simulink model "model_16_09_22"  (R2021a)
settings: Solver=FixedStepAuto  StartTime=0.0  StopTime=1370  FixedStep=0.01  RelTol=1e-3
values from neighbouring files (symbols this model uses):
  coord_0_ecef = [x_0_ecef, y_0_ecef, z_0_ecef]    [new_path_local_frame4_05_2022.m]
  dampPitchConst = 5    [Configuration_13_09_22FINESTRELLE.m]
  dampRollConst = 5    [Configuration_13_09_22FINESTRELLE.m]
  ECC = 0.0818191908426    [new_path_local_frame4_05_2022.m]
  FsGong = 8192    [matlabSounds.mat]
  FsHandel = 8192    [matlabSounds.mat]
  gainPitchTorque = -1000    [Configuration_13_09_22FINESTRELLE.m]
  gainRollTorque = -1000    [Configuration_13_09_22FINESTRELLE.m]
  indirect = 1    [Configuration_13_09_22FINESTRELLE.m]
  R_E = 6378137    [new_path_local_frame4_05_2022.m]
  RotationMatrix_NWU2ECEF = [-cos(lon0)*sin(lat0),  sin(lon0), cos(lon0)*cos(lat0) ... (first row only)    [new_path_local_frame4_05_2022.m]
  springPitchConst = 35    [Configuration_13_09_22FINESTRELLE.m]
  springRollConst = 35    [Configuration_13_09_22FINESTRELLE.m]
  timesPitch = 0.6    [Configuration_13_09_22FINESTRELLE.m]
  timesRoll = 0.6    [Configuration_13_09_22FINESTRELLE.m]
  yGong = [-0.00269844839217 -0.00449741398696 -0.00742073307848 -0.011018664268 -0.0128176298628 -0.0173150438498 -0.0222621992354 -0.0222621992354 -0.020013492242 -0.00921969867326 0.00449741398696 0.0101191814707 ... (42028 elements, 42028x1)]    [matlabSounds.mat]
  yHandel = [0 -0.00615680615681 -0.0750360750361 -0.0311688311688 0.00615680615681 0.0380952380952 0.0188552188552 -0.025012025012 -0.0311688311688 -0.0750360750361 -0.12582972583 -0.1443001443 ... (73113 elements, 73113x1)]    [matlabSounds.mat]
undefined symbols (not defined in the file or in its folder): DiscIntNeverNeededParam, f
libraries: cstblocks x7, simulink x6, instrumentlib x5
(part 1 of 2)
settings Model: SimulationMode=accelerator  Creator=vecluster  LastModifiedBy=LAR
settings SolverCC: AlgebraicLoopSolver=TrustRegion  MinimalZcImpactIntegration=on
settings DataIOCC: SaveFormat=StructureWithTime  SignalLoggingName=signals  ReturnWorkspaceOutputsName=ToWorkspace  LoggingToFile=on  LoggingFileName=logfile.mat
settings DebuggingCC: ArithmeticOperatorsInVariantConditions=warning
settings SFSimCC: CustomCodeUndefinedFunction=UseInterfaceOnly

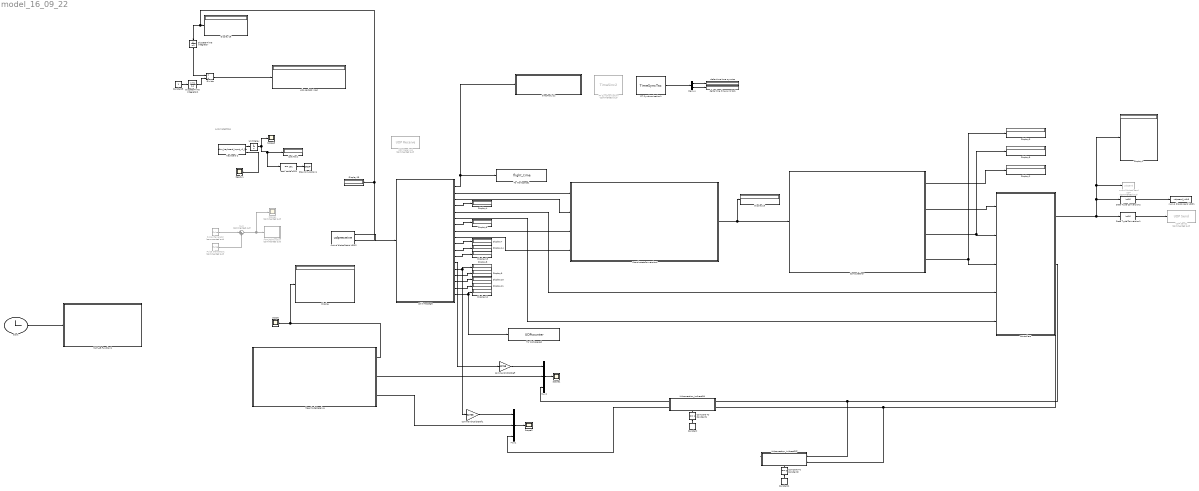
== system model_16_09_22 ==
  note: AutomatedStop
  Clock : Clock
  Compare To Constant1 : simulink/Logic and Bit Operations/Compare To Constant  relop===  const=1  OutDataTypeStr=boolean
  Compare To Constant2 : simulink/Logic and Bit Operations/Compare To Constant  relop===  const=0  OutDataTypeStr=boolean
  ComputeError : Subsystem
  Constant : Constant  Value=indirect  SampleTime=0.01
  Constant1 : Constant  Value=indirect  SampleTime=0.01
  Constant3 : Constant
  Controllers : Subsystem
  CoordinatesConversions : Subsystem
  Data Type Conversion1 : DataTypeConversion  OutDataTypeStr=int16
  Data Type Conversion2 : DataTypeConversion  OutDataTypeStr=int16
  Demux : Demux  Outputs=2
  Discrete-Time Integrator : DiscreteIntegrator  IntegratorMethod=Accumulation: Forward Euler  SampleTime=-1  ICPrevOutput=DiscIntNeverNeededParam  ICPrevScaledInput=DiscIntNeverNeededParam
  Discrete-Time Integrator1 : DiscreteIntegrator  InitialCondition=eps  SampleTime=-1  ICPrevOutput=DiscIntNeverNeededParam  ICPrevScaledInput=DiscIntNeverNeededParam
  Display{,1..16,23} (18 alike) : Display
  Divide : Product  Inputs=*/
  IHAcorrection_indirectON : Subsystem
  IHAcorrection_inidrectOFF : Subsystem
  Keyboard 2 : M-S-Function  FunctionName=sfun_keyboard_input_v1_2b  mask(Keyboard Input){}
      mask help: Keyboard Input
      mask Display: fprintf('Keyboard');
  Last Key1 : Display
  MATLAB Function : MATLAB Function  Commented=on  TreatAsAtomicUnit=on
  MATLAB Function1 : MATLAB Function  TreatAsAtomicUnit=on
  MagnitudeReceive : Subsystem
  Mux1 : Mux  Inputs=3
  Mux2 : Mux  Inputs=3
  Pulse Generator : DiscretePulseGenerator  Commented=on  PulseType=Time based  Period=1360  PulseWidth=0.01
  Pulse Generator1 : DiscretePulseGenerator  Commented=on  PulseType=Time based  Period=5  PulseWidth=0.1  PhaseDelay=1376
  RT Synchronization : S-Function  Commented=on  FunctionName=TimeSinc2  Parameters=st mf  SFunctionDeploymentMode=off  EnableBusSupport=off  mask(Pseudo-Real Time synchronization for Simulink Schemes){st=0.01, mf=200/140*200/255}
      mask prompts: st "Sample Time"; mf "Multiply factor"
      mask help:
      | This block synchronizes Simulink Simulation with RealTime.
      | The Real-Time versus Simulation-Time alignment is done every "Sample Time" seconds.
      | The Multiply Factor accelerates or slows real-Time: Multiply Factor=1 means real-time, Multiply Factor=2 means two times faster than real-time.
      | Use a Multiply Factor strictly > 0!!
      mask Display: disp(sprintf('RT Synchronization\n\nSample Time: %f\n Accelerator: %f',st,mf));
  RT Synchronization1 : S-Function  FunctionName=TimeSyncTsc  Parameters=st mf  SFunctionDeploymentMode=off  EnableBusSupport=off  mask(Pseudo-Real Time synchronization for Simulink Schemes){st=0.01, mf=1}
      mask prompts: st "Sample Time"; mf "Multiply factor"
      mask help:
      | This block synchronizes Simulink Simulation with RealTime.
      | The Real-Time versus Simulation-Time alignment is done every "Sample Time" seconds.
      | The Multiply Factor accelerates or slows real-Time: Multiply Factor=1 means real-time, Multiply Factor=2 means two times faster than real-time.
      | Use a Multiply Factor strictly > 0!!
      mask Display: disp(sprintf('RT Synchronization\n\nSample Time: %f\n Accelerator: %f',st,mf));
  Ready1 : Scope
  Scope{,1..3} (4 alike) : Scope
  Scope4 : Scope  Commented=on
  Stop Simulation1 : Stop
  Sum : Sum  Commented=on  Inputs=|++
  To Workspace1 : ToWorkspace  VariableName=flight_time  SaveFormat=Structure With Time  SampleTime=-1
  To Workspace2 : ToWorkspace  VariableName=UDPcounter  SaveFormat=Structure With Time  SampleTime=-1
  UDP Receive1 : instrumentlib/UDP Receive  Commented=on  Host=0.0.0.0  Port=1  LocalPort=6060  EnablePortSharing=on  GetLatestData=on  DataSize="[20   1]"  DataType=double  ASCIIFormatting=%f,  Terminator=LF  ByteOrder=LittleEndian  EnableBlockingMode=off  Timeout=100  SampleTime=0.01  LocalAddress=127.0.0.1
  UDP Send1 : instrumentlib/UDP Send  Commented=on  Host=192.168.51.103  Port=5347  LocalPort=-1  EnablePortSharing=on  ByteOrder=LittleEndian  OutputDatagramPacketSize=24  EnableBlockingMode=off  LocalAddress=0.0.0.0
  Unit Delay : UnitDelay  SampleTime=0.1  HasFrameUpgradeWarning=on
  ascii code of E1 : simulink/Logic and Bit Operations/Compare To Constant  relop===  const=101  OutDataTypeStr=boolean
  commandXstickDefl : Gain  Gain=32768
  commandXstickDefl1 : Gain  Gain=32768
  delta time time sync tsc : Display
  delta time time sync tsc1 : Display
  nuovo blocco send UDP : S-Function  Commented=on  FunctionName=udpsend  Parameters='127.0.0.1','192.168.51.103', 55555, 0.01  SFunctionDeploymentMode=off  EnableBusSupport=off
  nuovo blocco send UDP1 : S-Function  FunctionName=udpsend_int16  Parameters='127.0.0.1','192.168.51.103', 5347, 0.01  SFunctionDeploymentMode=off  EnableBusSupport=off
  nuovo blocco send UDP2 : S-Function  FunctionName=udpreceive  Parameters='127.0.0.1', 6060, 0.01, 20  SFunctionDeploymentMode=off  EnableBusSupport=off
  split message : MATLAB Function  TreatAsAtomicUnit=on
  timeAnalysis : Subsystem
  udp packets / sec : Display
  wires:
  Data Type Conversion1/1 -> UDP Send1/1  "StickCmd_INT16"
  CoordinatesConversions/1(plane_coord_nwu) -> Display23/1, ComputeError/1(plane_coord_nwu)  "plane_coord_nwu"
  split message/2(lat) -> CoordinatesConversions/1(lat)  "latRad"
  split message/3(lon) -> CoordinatesConversions/2(lon)  "lonRad"
  split message/8(coord_ecef_aerofly) -> CoordinatesConversions/3(aeroflyECEF)  "aeroflyECEF"
  split message/9(altitude) -> CoordinatesConversions/4(alt)  "altitude"
  ComputeError/2(intersection2path) -> Controllers/1(intesection2path)  "intesection2path"
  ComputeError/3(h) -> Display5/1, Controllers/2(h)  "h"
  ComputeError/4(s) -> Display3/1, Controllers/3(s)  "s"
  split message/5(roll) -> Controllers/4(rollAngle)  "roll"
  ComputeError/1(min_valid_index) -> Display2/1  "min_valid_index"
  Controllers/1(dataSend) -> Data Type Conversion2/1, nuovo blocco send UDP/1, Display1/1, Data Type Conversion1/1  "DataSend"
  split message/1(flight_time) -> timeAnalysis/1(flightTime), To Workspace1/1  "flightTime"
  split message/4(height) -> Display4/1  "height"
  split message/7(yaw) -> Display6/1  "yaw"
  split message/18(UDPcounter) -> Display12/1, To Workspace2/1  "UDPcounter"
  split message/14(aircraft_elevator) -> Display8/1, commandXstickDefl1/1  "elevator"
  split message/10(controls_roll_input) -> Display7/1  "control_roll_in"
  split message/11(controls_pitch_input) -> Display14/1  "control_pitch_in"
  split message/12(controls_yaw_input) -> Display13/1  "control_yaw_in"
  split message/6(pitch) -> Controllers/5(pitch)  "pitch"
  split message/15(aircraft_velocityX) -> Display9/1  "aircraftVelX"
  split message/16(aircraft_velocityY) -> Display10/1  "aircraftVelY"
  split message/17(aircraft_velocityZ) -> Display11/1  "aircraftVelZ"
  Mux2/1 -> Scope1/1
  commandXstickDefl/1 -> Mux2/1  "fromAileron2Command"
  Controllers/2(trimCorrectionRoll) -> IHAcorrection_inidrectOFF/1(trimCorrectionRoll), IHAcorrection_indirectON/1(trimCorrectionRoll)  "trimCorrectionsRoll"
  Controllers/3(trimCorrectionPitch) -> IHAcorrection_inidrectOFF/2(trimCorrectionPitch), IHAcorrection_indirectON/2(trimCorrectionPitch)  "trimCorrectionsPitch"
  IHAcorrection_indirectON/1(iha_correction_rollToSend) -> Mux2/3  "ihaCorrectionRollMagnitude"
  MagnitudeReceive/1(stickDeflectionVectorScaled) -> Display/1, Scope/1
  MagnitudeReceive/2(StickDeflRollReceived) -> Mux2/2  "StickDeflRollReceived"
  Constant/1 -> Compare To Constant1/1  "indirectON"
  Compare To Constant1/1 -> IHAcorrection_indirectON/Enable
  split message/13(aircraft_aileron) -> commandXstickDefl/1  "aileron"
  commandXstickDefl1/1 -> Mux1/1  "fromElevator2Command"
  MagnitudeReceive/3(StickDeflPitchReceived) -> Mux1/2  "StickDeflPitchReceived"
  IHAcorrection_indirectON/2(iha_correction_pitchToSend) -> Mux1/3  "ihaCorrectionPitchMagnitude"
  Mux1/1 -> Scope2/1
  Compare To Constant2/1 -> IHAcorrection_inidrectOFF/Enable
  Constant1/1 -> Compare To Constant2/1  "indirectOFF"
  IHAcorrection_inidrectOFF/1(iha_correction_rollToSend) -> ?
  Sum/1 -> MATLAB Function/1(start), Scope4/1  "audio"
  Pulse Generator1/1 -> Sum/2
  Pulse Generator/1 -> Sum/1
  ascii code of E1/1 -> Stop Simulation1/1
  Keyboard 2/2 -> Ready1/1
  Keyboard 2/1 -> Unit Delay/1
  RT Synchronization1/1 -> Demux/1  "TimeSyncTsc_output"
  Demux/1 -> delta time time sync tsc/1
  Unit Delay/1 -> ascii code of E1/1, Last Key1/1, Scope3/1
  nuovo blocco send UDP2/1 -> split message/1(u)  "UDPreceiveAerofly"
  nuovo blocco send UDP2/2 -> Discrete-Time Integrator/1, Display16/1, Display15/1  "UDPreceive1status"
  Discrete-Time Integrator/1 -> Divide/1
  Discrete-Time Integrator1/1 -> Divide/2
  Constant3/1 -> Discrete-Time Integrator1/1
  Divide/1 -> udp packets / sec/1  "packetsXsecondUDPreceive1"
  Demux/2 -> delta time time sync tsc1/1
  Data Type Conversion2/1 -> nuovo blocco send UDP1/1  "StickCmd_INT16"
  Clock/1 -> MATLAB Function1/1(start)  "simtime"

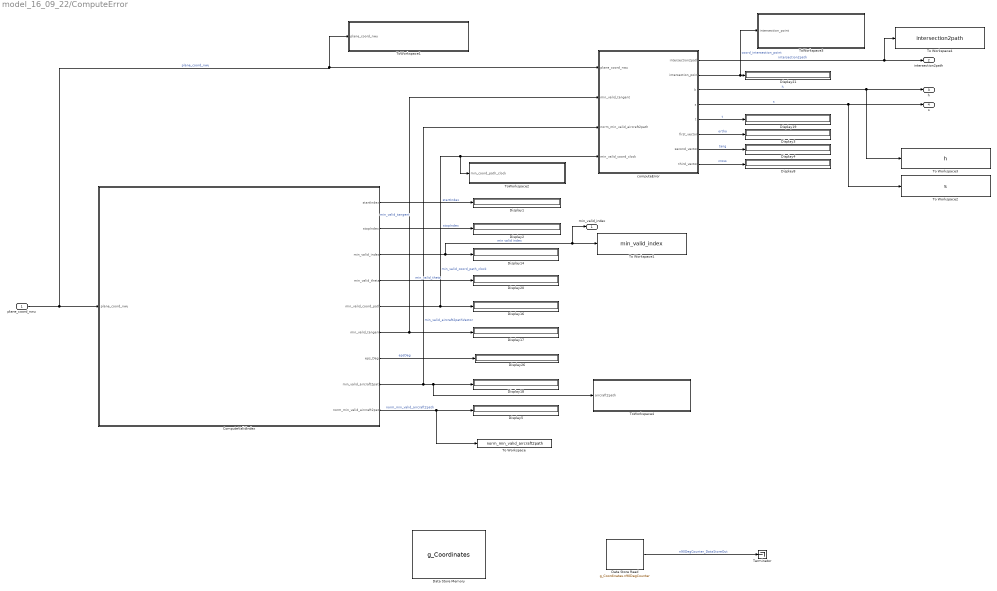
== system model_16_09_22/ComputeError ==
  plane_coord_nwu : Inport
  ComputeValidIndex : MATLAB Function  TreatAsAtomicUnit=on
  Data Store Memory : DataStoreMemory  DataStoreName=g_Coordinates  ReadBeforeWriteMsg=warning  WriteAfterWriteMsg=warning  WriteAfterReadMsg=warning  InitialValue=coord_clock_Struct  ShowAdditionalParam=off  OutDataTypeStr=Bus: ExperimentConfigAerofly
  Data Store Read : DataStoreRead  DataStoreName=g_Coordinates  DataStoreElements=g_Coordinates.n90DegCounter  IndexOptions=Index vector (dialog)  Indices=1  OutputSizes=1
  Display{1..5,8,14,16..21,26} (14 alike) : Display
  Terminator : Terminator
  To Workspace : ToWorkspace  VariableName=norm_min_valid_aircraft2path  SaveFormat=Structure With Time  SampleTime=-1
  To Workspace1 : ToWorkspace  VariableName=min_valid_index  SaveFormat=Structure With Time  SampleTime=-1
  To Workspace2 : ToWorkspace  VariableName=s  SaveFormat=Structure With Time  SampleTime=-1
  To Workspace3 : ToWorkspace  VariableName=h  SaveFormat=Structure With Time  SampleTime=-1
  To Workspace4 : ToWorkspace  VariableName=intersection2path  SaveFormat=Structure With Time  SampleTime=-1
  ToWorkspace1 : Subsystem
  ToWorkspace2 : Subsystem
  ToWorkspace3 : Subsystem
  ToWorkspace4 : Subsystem
  computeError : MATLAB Function  TreatAsAtomicUnit=on
  min_valid_index : Outport
  intersection2path : Outport  Port=2
  h : Outport  Port=3
  s : Outport  Port=4
  wires:
  computeError/1(intersection2path) -> To Workspace4/1, intersection2path/1  "intersection2path"
  ComputeValidIndex/7(eps_Deg) -> Display26/1  "epsDeg"
  computeError/6(first_vector) -> Display3/1  "ortho"
  ComputeValidIndex/4(min_valid_theta) -> Display20/1  "min_valid_theta"
  computeError/8(third_vector) -> Display8/1  "cross"
  computeError/7(second_vector) -> Display4/1  "tang"
  ComputeValidIndex/8(min_valid_aircraft2path) -> computeError/3(norm_min_valid_aircraft2path), ToWorkspace4/1(aircraft2path), Display18/1  "min_valid_aircraft2pathVector"
  ComputeValidIndex/6(min_valid_tangent) -> computeError/2(min_valid_tangent), Display17/1  "min_valid_tangent"
  computeError/5(t) -> Display19/1  "t"
  ComputeValidIndex/5(min_valid_coord_path) -> ToWorkspace2/1(min_coord_path_clock), computeError/4(min_valid_coord_clock), Display16/1  "min_valid_coord_path_clock"
  ComputeValidIndex/2(stopIndex) -> Display2/1  "stopIndex"
  computeError/2(intersection_point) -> ToWorkspace3/1(intersection_point), Display21/1  "coord_intersection_point"
  ComputeValidIndex/1(startIndex) -> Display1/1  "startIndex"
  ComputeValidIndex/3(min_valid_index) -> min_valid_index/1, To Workspace1/1, Display14/1  "min valid index"
  ComputeValidIndex/9(norm_min_valid_aircraft2path) -> Display5/1, To Workspace/1  "norm_min_valid_aircraft2path"
  Data Store Read/1 -> Terminator/1  "n90DegCounter_DataStoreOut"
  computeError/3(h) -> h/1, To Workspace3/1  "h"
  computeError/4(s) -> To Workspace2/1, s/1  "s"
  plane_coord_nwu/1 -> ComputeValidIndex/1(plane_coord_nwu), ToWorkspace1/1(plane_coord_nwu), computeError/1(plane_coord_nwu)  "plane_coord_nwu"

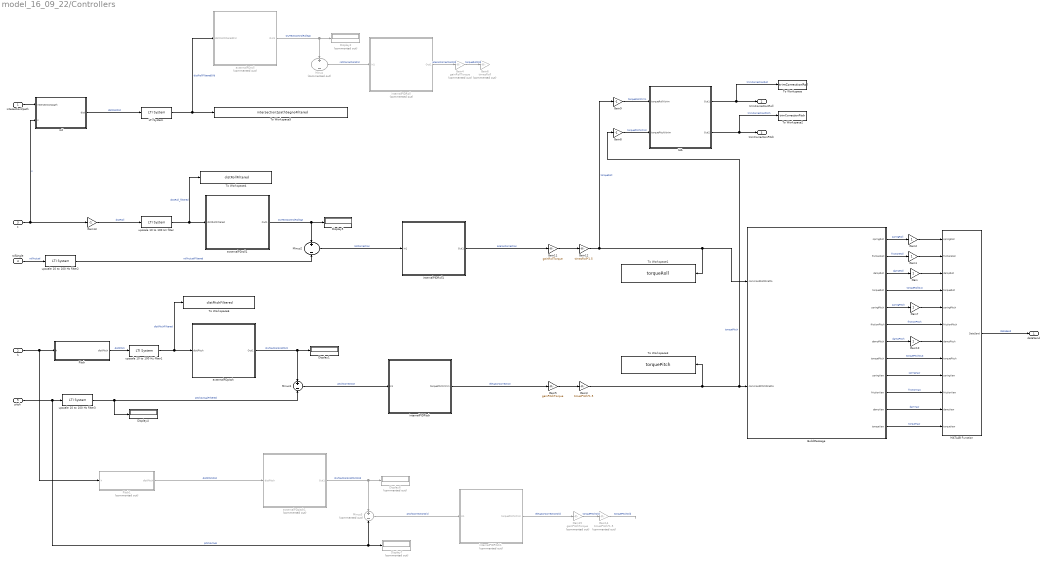
== system model_16_09_22/Controllers ==
  intesection2path : Inport
  h : Inport  Port=2
  s : Inport  Port=3
  rollAngle : Inport  Port=4
  pitch : Inport  Port=5
  BuildMessage : MATLAB Function  TreatAsAtomicUnit=on
  Display1 : Display
  Display2 : Display  Commented=on
  Display4 : Display
  Display5 : Display
  Display6 : Display  Commented=on
  Display7 : Display  Commented=on
  Gain{,1..2,7,10} (5 alike) : Gain
  Gain11 : Gain  Gain=gainRollTorque
  Gain12 : Gain  Gain=timesRoll*1.5
  Gain13 : Gain  Gain=-1
  Gain14 : Gain  Commented=on  Gain=timesPitch*1.5
  Gain15 : Gain  Commented=on  Gain=gainPitchTorque
  Gain3 : Gain  Gain=timesPitch*1.5
  Gain4 : Gain  Commented=on  Gain=gainRollTorque
  Gain5 : Gain  Gain=gainPitchTorque
  Gain6 : Gain  Commented=on  Gain=timesRoll
  Gain8 : Gain  Gain=-1
  Gain9 : Gain  Gain=-1
  IHA : Subsystem  TreatAsAtomicUnit=on
  LTI System : cstblocks/LTI System  sys=FILTER01  IC=[]
  MATLAB Function : MATLAB Function  TreatAsAtomicUnit=on
  Minus : Sum  Commented=on  Inputs=+-
  Minus1 : Sum  Inputs=+-
  Minus2 : Sum  Inputs=+-
  Minus3 : Sum  Commented=on  Inputs=+-
  Pitch : MATLAB Function  TreatAsAtomicUnit=on
  Pitch1 : MATLAB Function  Commented=on  TreatAsAtomicUnit=on
  To Workspace : ToWorkspace  VariableName=trimCorrectionRoll  SaveFormat=Structure With Time  SampleTime=-1
  To Workspace1 : ToWorkspace  VariableName=torqueRoll  SaveFormat=Structure With Time  SampleTime=-1
  To Workspace2 : ToWorkspace  VariableName=trimCorrectionPitch  SaveFormat=Structure With Time  SampleTime=-1
  To Workspace3 : ToWorkspace  VariableName=torquePitch  SaveFormat=Structure With Time  SampleTime=-1
  To Workspace4 : ToWorkspace  VariableName=distRollFiltered  SaveFormat=Structure With Time  SampleTime=-1
  To Workspace5 : ToWorkspace  VariableName=intersection2pathSegnoFiltered  SaveFormat=Structure With Time  SampleTime=-1
  To Workspace6 : ToWorkspace  VariableName=distPitchFiltered  SaveFormat=Structure With Time  SampleTime=-1
  externalPDpitch : Subsystem
  externalPDpitch1 : Subsystem  Commented=on
  externalPDroll : Subsystem  Commented=on
  externalPDroll1 : Subsystem
  internalPIDPitch : Subsystem
  internalPIDPitch1 : Subsystem  Commented=on
  internalPIDRoll : Subsystem  Commented=on
  internalPIDRoll1 : Subsystem
  roll : MATLAB Function  TreatAsAtomicUnit=on
  upscale 10 to 100 Hz filter{,1..3} (4 alike) : cstblocks/LTI System  sys=FILTER02  IC=[]
  dataSend : Outport
  trimCorrectionRoll : Outport  Port=2
  trimCorrectionPitch : Outport  Port=3
  wires:
  h/1 -> Pitch1/1(h), Pitch/1(h)
  s/1 -> Gain13/1, roll/2(s)  "s"
  Minus/1 -> internalPIDRoll/1(In1)  "rollCorrectionOld"
  Minus1/1 -> internalPIDPitch/1(In1)  "pitchCorrection"
  internalPIDPitch/1(torquePitchXtrim) -> Gain5/1  "elevatorCorrection"
  externalPDpitch/1(Out1) -> Display1/1, Minus1/1  "OUTextControlPitch"
  internalPIDRoll/1(Out1) -> Gain4/1  "aileronCorrectionOld"
  MATLAB Function/1(DataSend) -> dataSend/1  "DataSend"
  BuildMessage/3(dampRoll) -> Gain/1  "dampRoll"
  BuildMessage/4(torqueRoll) -> MATLAB Function/4(torqueRoll)  "torqueRollOut"
  BuildMessage/5(springPitch) -> Gain7/1  "springPitch"
  BuildMessage/6(frictionPitch) -> MATLAB Function/6(frictionPitch)  "frictionPitch"
  BuildMessage/7(dampPitch) -> Gain10/1  "dampPitch"
  BuildMessage/8(torquePitch) -> MATLAB Function/8(torquePitch)  "torquePitchOut"
  BuildMessage/9(springYaw) -> MATLAB Function/9(springYaw)  "springYaw"
  BuildMessage/10(frictionYaw) -> MATLAB Function/10(frictionYaw)  "frictionYaw"
  BuildMessage/11(dampYaw) -> MATLAB Function/11(dampYaw)  "damYaw"
  BuildMessage/12(torqueYaw) -> MATLAB Function/12(torqueYaw)  "torqueYaw"
  Pitch/1(distPitch) -> upscale 10 to 100 Hz filter1/1  "distPitch"
  externalPDroll/1(Out1) -> Minus/1, Display2/1  "OUTextControlRollSat"
  roll/1(dist) -> LTI System/1  "distRollOld"
  BuildMessage/2(frictionRoll) -> Gain1/1  "frictionRoll"
  BuildMessage/1(springRoll) -> Gain2/1  "springRoll"
  IHA/1(Out1) -> To Workspace/1, trimCorrectionRoll/1  "trimCorrectionRoll"
  IHA/2(Out2) -> trimCorrectionPitch/1, To Workspace2/1  "trimCorrectionPitch"
  Gain4/1 -> Gain6/1  "torqueRollOld"
  Gain5/1 -> Gain3/1
  Gain1/1 -> MATLAB Function/2(frictionRoll)
  Gain/1 -> MATLAB Function/3(dampRoll)
  Gain2/1 -> MATLAB Function/1(springRoll)
  Gain3/1 -> To Workspace3/1, BuildMessage/2(commandPitchDiretto), Gain8/1  "torquePitch"
  Gain7/1 -> MATLAB Function/5(springPitch)
  Gain9/1 -> IHA/1(torqueRollXtrim)  "torqueRollXtrim"
  Gain8/1 -> IHA/2(torquePitchXtrim)  "torquePitchXtrim"
  Gain10/1 -> MATLAB Function/7(dampPitch)
  LTI System/1 -> externalPDroll/1(distRollFilteredOld), To Workspace5/1  "distRollFilteredOld"
  externalPDroll1/1(Out1) -> Display5/1, Minus2/1  "OUTextControlRollSat"
  internalPIDRoll1/1(Out1) -> Gain11/1  "aileronCorrection"
  Minus2/1 -> internalPIDRoll1/1(In1)  "rollCorrection"
  rollAngle/1 -> upscale 10 to 100 Hz filter2/1  "rollActual"
  Gain11/1 -> Gain12/1
  Gain12/1 -> BuildMessage/1(commandRollDiretto), To Workspace1/1, Gain9/1  "torqueRoll"
  Gain13/1 -> upscale 10 to 100 Hz filter/1  "distRoll"
  upscale 10 to 100 Hz filter/1 -> To Workspace4/1, externalPDroll1/1(distRollFiltered)  "distRoll_fIltered"
  upscale 10 to 100 Hz filter2/1 -> Minus2/2  "rollActualFiltered"
  upscale 10 to 100 Hz filter1/1 -> To Workspace6/1, externalPDpitch/1(distPitch)  "distPitchFiltered"
  upscale 10 to 100 Hz filter3/1 -> Minus1/2, Display4/1  "pitchActualFiltered"
  externalPDpitch1/1(Out1) -> Display6/1, Minus3/1  "OUTextControlPitchOld"
  Minus3/1 -> internalPIDPitch1/1(In1)  "pitchCorrectionOld"
  internalPIDPitch1/1(torquePitchXtrim) -> Gain15/1  "elevatorCorrectionOld"
  pitch/1 -> upscale 10 to 100 Hz filter3/1, Minus3/2, Display7/1  "pitchActual"
  Pitch1/1(distPitch) -> externalPDpitch1/1(distPitch)  "distPitchOld"
  Gain14/1 -> ?  "torquePitchOld"
  Gain15/1 -> Gain14/1  "torquePitchOld"
  intesection2path/1 -> roll/1(intersection2path)

== system model_16_09_22/CoordinatesConversions ==
  note: HO MESSO LE COORD LOCALI DIPENDENTI DALL'ECEF DI AEROFLY PER EVITARE DI AGGIUNGERE ERRORI DOVUTI ALLE MIE MATRICI DI ROTAZIONE DA LON LAT AD ECEF
  lat : Inport
  lon : Inport  Port=2
  aeroflyECEF : Inport  Port=3
  alt : Inport  Port=4
  Display{,1..2,7,24..25} (6 alike) : Display
  MATLAB Function : MATLAB Function  TreatAsAtomicUnit=on
  MATLAB Function2 : MATLAB Function  TreatAsAtomicUnit=on
  MATLAB Function3 : MATLAB Function  TreatAsAtomicUnit=on
  plane_coord_nwu : Outport
  wires:
  MATLAB Function3/1(lonDeg) -> Display24/1  "lonDeg"
  MATLAB Function/1(coord_ecef) -> Display/1, MATLAB Function2/1(coord_ecef)  "myECEF"
  aeroflyECEF/1 -> Display7/1, MATLAB Function2/2(coord_ecef_aerofly)  "aeroflyECEF"
  MATLAB Function2/1(plane_coord_nwu) -> Display2/1  "plane_coord_nwu_myECEF"
  MATLAB Function3/2(latDeg) -> Display25/1  "latDeg"
  lon/1 -> MATLAB Function3/1(lon), MATLAB Function/2(lon)
  lat/1 -> MATLAB Function3/2(lat), MATLAB Function/1(lat)
  alt/1 -> MATLAB Function2/3(alt), MATLAB Function/3(alt)  "altitude"
  MATLAB Function2/2(plane_coord_nwu_aerofly) -> Display1/1, plane_coord_nwu/1  "plane_coord_nwu_aeroflyECEF"

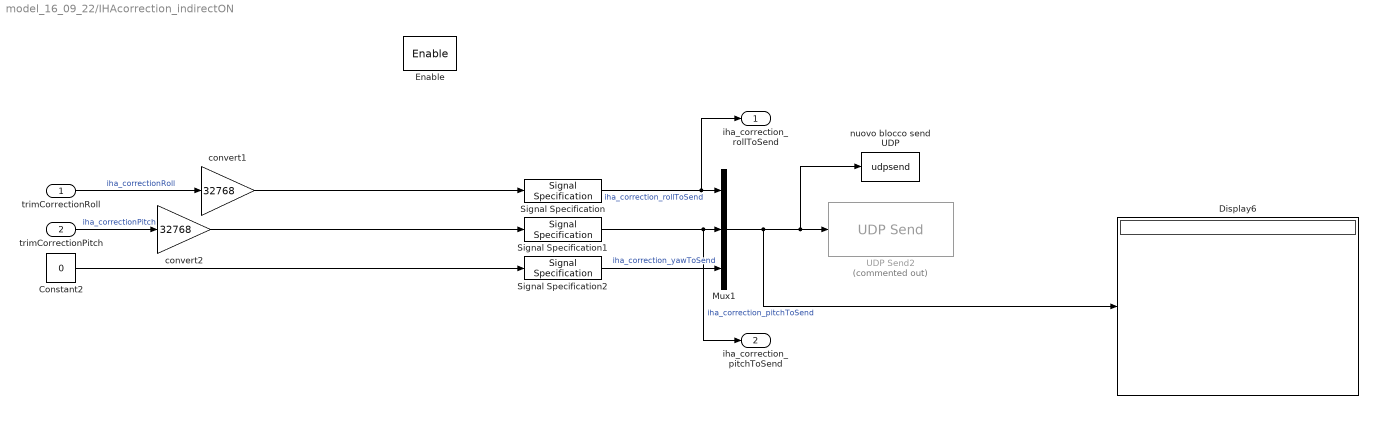
== system model_16_09_22/IHAcorrection_indirectON ==
  trimCorrectionRoll : Inport
  trimCorrectionPitch : Inport  Port=2
  Enable : EnablePort
  Constant2 : Constant  Value=0  SampleTime=0.01
  Display6 : Display
  Mux1 : Mux  Inputs=3
  Signal Specification : SignalSpecification  OutDataTypeStr=double  Dimensions=1
  Signal Specification1 : SignalSpecification  OutDataTypeStr=double  Dimensions=1
  Signal Specification2 : SignalSpecification  OutDataTypeStr=double  Dimensions=1
  UDP Send2 : instrumentlib/UDP Send  Commented=on  Host=127.0.0.1  Port=25346  LocalPort=-1  EnablePortSharing=on  ByteOrder=LittleEndian  OutputDatagramPacketSize=24  EnableBlockingMode=off  LocalAddress=0.0.0.0
  convert1 : Gain  Gain=32768
  convert2 : Gain  Gain=32768
  nuovo blocco send UDP : S-Function  FunctionName=udpsend  Parameters='127.0.0.1','127.0.0.1', 25346, 0.01  SFunctionDeploymentMode=off  EnableBusSupport=off
  iha_correction_rollToSend : Outport
  iha_correction_pitchToSend : Outport  Port=2
  wires:
  Signal Specification/1 -> iha_correction_rollToSend/1, Mux1/1  "iha_correction_rollToSend"
  Signal Specification1/1 -> iha_correction_pitchToSend/1, Mux1/2  "iha_correction_pitchToSend"
  Signal Specification2/1 -> Mux1/3  "iha_correction_yawToSend"
  Mux1/1 -> Display6/1, nuovo blocco send UDP/1, UDP Send2/1
  convert2/1 -> Signal Specification1/1
  Constant2/1 -> Signal Specification2/1
  convert1/1 -> Signal Specification/1
  trimCorrectionRoll/1 -> convert1/1  "iha_correctionRoll"
  trimCorrectionPitch/1 -> convert2/1  "iha_correctionPitch"

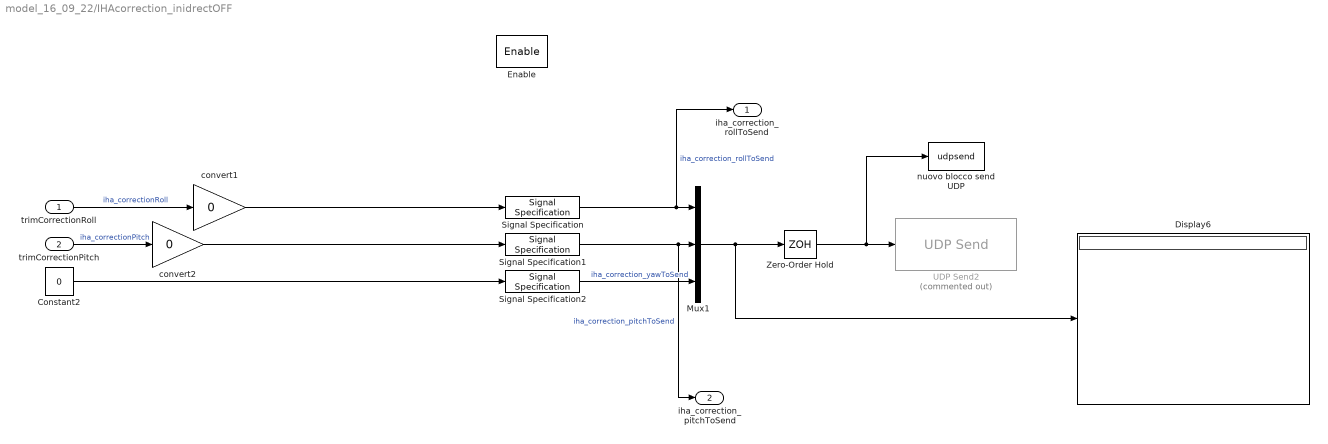
== system model_16_09_22/IHAcorrection_inidrectOFF ==
  trimCorrectionRoll : Inport
  trimCorrectionPitch : Inport  Port=2
  Enable : EnablePort
  Constant2 : Constant  Value=0  SampleTime=0.01
  Display6 : Display
  Mux1 : Mux  Inputs=3
  Signal Specification : SignalSpecification  OutDataTypeStr=double  Dimensions=1
  Signal Specification1 : SignalSpecification  OutDataTypeStr=double  Dimensions=1
  Signal Specification2 : SignalSpecification  OutDataTypeStr=double  Dimensions=1
  UDP Send2 : instrumentlib/UDP Send  Commented=on  Host=127.0.0.1  Port=25346  LocalPort=-1  EnablePortSharing=on  ByteOrder=LittleEndian  OutputDatagramPacketSize=24  EnableBlockingMode=off  LocalAddress=0.0.0.0
  Zero-Order Hold : ZeroOrderHold  SampleTime=0.01
  convert1 : Gain  Gain=0
  convert2 : Gain  Gain=0
  nuovo blocco send UDP : S-Function  FunctionName=udpsend  Parameters='127.0.0.1','127.0.0.1', 25346, 0.01  SFunctionDeploymentMode=off  EnableBusSupport=off
  iha_correction_rollToSend : Outport
  iha_correction_pitchToSend : Outport  Port=2
  wires:
  trimCorrectionPitch/1 -> convert2/1  "iha_correctionPitch"
  trimCorrectionRoll/1 -> convert1/1  "iha_correctionRoll"
  convert1/1 -> Signal Specification/1
  convert2/1 -> Signal Specification1/1
  Constant2/1 -> Signal Specification2/1
  Mux1/1 -> Display6/1, Zero-Order Hold/1
  Signal Specification1/1 -> iha_correction_pitchToSend/1, Mux1/2  "iha_correction_pitchToSend"
  Signal Specification2/1 -> Mux1/3  "iha_correction_yawToSend"
  Signal Specification/1 -> iha_correction_rollToSend/1, Mux1/1  "iha_correction_rollToSend"
  Zero-Order Hold/1 -> nuovo blocco send UDP/1, UDP Send2/1

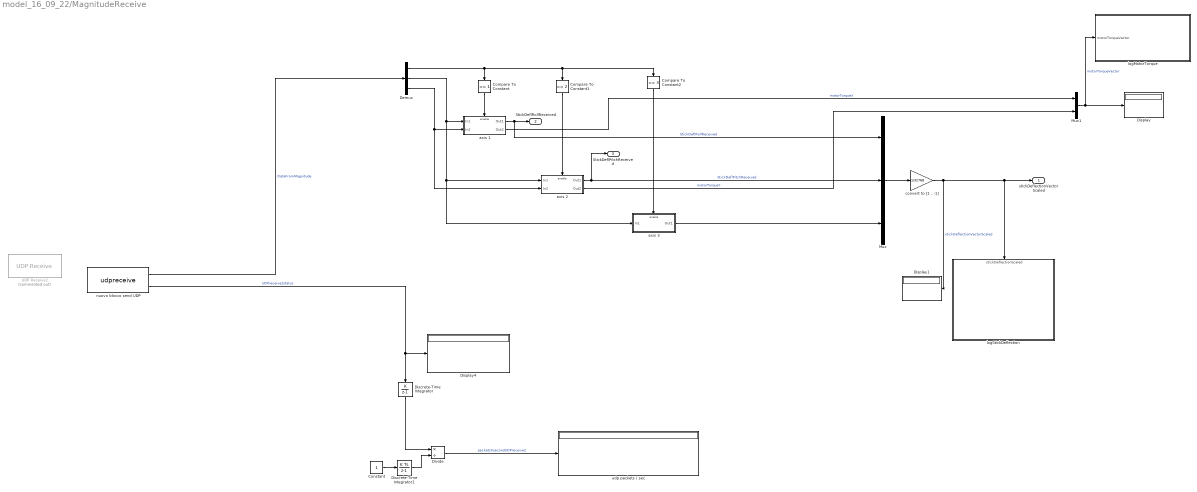
== system model_16_09_22/MagnitudeReceive ==
  Compare To Constant : simulink/Logic and Bit Operations/Compare To Constant  relop===  const=1  OutDataTypeStr=boolean
  Compare To Constant1 : simulink/Logic and Bit Operations/Compare To Constant  relop===  const=2  OutDataTypeStr=boolean
  Compare To Constant2 : simulink/Logic and Bit Operations/Compare To Constant  relop===  const=3  OutDataTypeStr=boolean
  Constant : Constant
  Demux : Demux  Outputs=3
  Discrete-Time Integrator : DiscreteIntegrator  IntegratorMethod=Accumulation: Forward Euler  SampleTime=-1  ICPrevOutput=DiscIntNeverNeededParam  ICPrevScaledInput=DiscIntNeverNeededParam
  Discrete-Time Integrator1 : DiscreteIntegrator  InitialCondition=eps  SampleTime=-1  ICPrevOutput=DiscIntNeverNeededParam  ICPrevScaledInput=DiscIntNeverNeededParam
  Display : Display
  Display1 : Display
  Display4 : Display
  Divide : Product  Inputs=*/
  Mux : Mux  Inputs=3
  Mux1 : Mux  Inputs=2
  UDP Receive2 : instrumentlib/UDP Receive  Commented=on  Host=0.0.0.0  Port=1  LocalPort=15346  EnablePortSharing=on  GetLatestData=on  DataSize="[3  1]"  DataType=double  ASCIIFormatting=%f,  Terminator=LF  ByteOrder=LittleEndian  EnableBlockingMode=off  Timeout=100  SampleTime=0.01  LocalAddress=192.168.51.167
  axis 1 : Subsystem  TreatAsAtomicUnit=on
  axis 2 : Subsystem  TreatAsAtomicUnit=on
  axis 3 : Subsystem  TreatAsAtomicUnit=on
  "convert to [1 , -1]" : Gain  Gain=1/32768
  logMotorTorque : Subsystem
  logStickDeflection : Subsystem
      settings: PortSchema="{\"entries\":[{\"content\":{\"sides\":[{\"content\":{\"connectorIds\":[]},\"type\":\"ConnectorPlacement.EquallySpacedRectSide\",\"uuid\":\"5b9206d2-2bc2-4e28-a507-3ced3b2864fd\"},{\"content\":{\"connectorIds\":[],\"side\":\"RIGHT\"},\"type\":\"ConnectorPlacement.EquallySpacedRectSide\",\"uuid\":\"17cd0793-c180-4ecb-a30b-5686e76381ab\"},{\"content\":{\"connectorIds\":[\"In1\"],\"side\":\"TOP\"},\"type\":\"ConnectorPlacement.EquallySpacedRectSide\",\"uuid\":\"03f68054-5148-47f9-aa1c-f06d50213310\"}]},\"type\":\"ConnectorPlacement.EquallySpacedConnector\",\"uuid\":\"762bc23e-4407-48eb-ab87-0feabf7a8a60\"}],\"packageUris\":[\"http://schema.mathworks.com/mf0/Connector/R2020b\"],\"version\":\"1.0\"}"
  nuovo blocco send UDP : S-Function  FunctionName=udpreceive  Parameters='192.168.51.167', 15346, 0.01, 3  SFunctionDeploymentMode=off  EnableBusSupport=off
  udp packets / sec : Display
  stickDeflectionVectorScaled : Outport
  StickDeflRollReceived : Outport  Port=2
  StickDeflPitchReceived : Outport  Port=3
  wires:
  Demux/1 -> Compare To Constant2/1, Compare To Constant1/1, Compare To Constant/1
  axis 1/1(Out1) -> Mux/1, StickDeflRollReceived/1  "StickDeflRollReceived"
  "convert to [1 , -1]"/1 -> Display1/1, logStickDeflection/1(stickDeflectionScaled), stickDeflectionVectorScaled/1  "stickDeflectionVectorScaled"
  Compare To Constant1/1 -> axis 2/Enable
  nuovo blocco send UDP/2 -> Discrete-Time Integrator/1, Display4/1  "UDPreceive2status"
  axis 3/1(Out1) -> Mux/3
  Compare To Constant/1 -> axis 1/Enable
  axis 2/1(Out1) -> StickDeflPitchReceived/1, Mux/2  "StickDeflPitchReceived"
  Divide/1 -> udp packets / sec/1  "packetsXsecondUDPreceive2"
  Discrete-Time Integrator1/1 -> Divide/2
  Discrete-Time Integrator/1 -> Divide/1
  Compare To Constant2/1 -> axis 3/Enable
  Mux/1 -> "convert to [1 , -1]"/1
  Constant/1 -> Discrete-Time Integrator1/1
  axis 1/2(Out2) -> Mux1/1  "motorTorqueX"
  axis 2/2(Out2) -> Mux1/2  "motorTorqueY"
  Mux1/1 -> Display/1, logMotorTorque/1(motorTorqueVector)  "motorTorqueVector"
  nuovo blocco send UDP/1 -> Demux/1  "DataFromMagnitude"
  Demux/2 -> axis 3/1(In1), axis 2/1(In1), axis 1/1(In1)
  Demux/3 -> axis 2/2(In2), axis 1/2(In2)

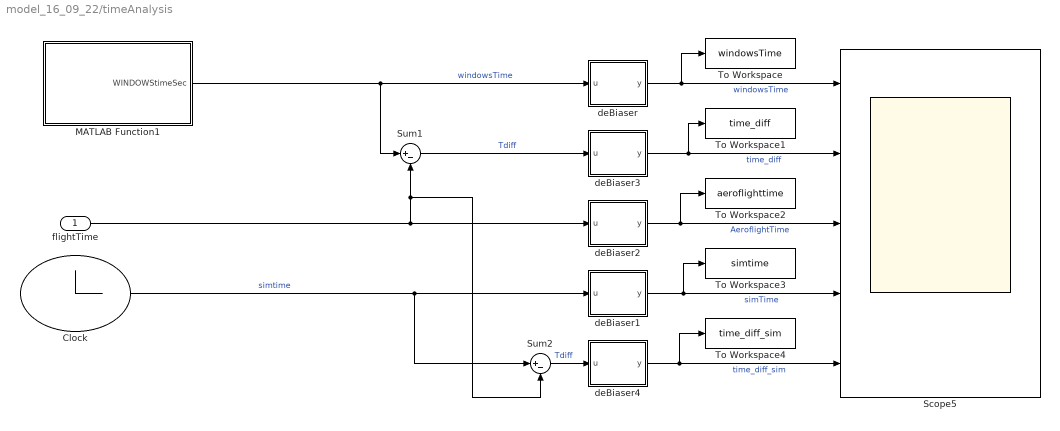
== system model_16_09_22/timeAnalysis ==
  flightTime : Inport
  Clock : Clock
  MATLAB Function1 : MATLAB Function  TreatAsAtomicUnit=on
  Scope5 : Scope  NumInputPorts=5
  Sum1 : Sum  Inputs=|+-
  Sum2 : Sum  Inputs=|+-
  To Workspace : ToWorkspace  VariableName=windowsTime  SaveFormat=Timeseries  SampleTime=-1
  To Workspace1 : ToWorkspace  VariableName=time_diff  SaveFormat=Timeseries  SampleTime=-1
  To Workspace2 : ToWorkspace  VariableName=aeroflighttime  SaveFormat=Timeseries  SampleTime=-1
  To Workspace3 : ToWorkspace  VariableName=simtime  SaveFormat=Timeseries  SampleTime=-1
  To Workspace4 : ToWorkspace  VariableName=time_diff_sim  SaveFormat=Timeseries  SampleTime=-1
  deBiaser : MATLAB Function  TreatAsAtomicUnit=on
  deBiaser1 : MATLAB Function  TreatAsAtomicUnit=on
  deBiaser2 : MATLAB Function  TreatAsAtomicUnit=on
  deBiaser3 : MATLAB Function  TreatAsAtomicUnit=on
  deBiaser4 : MATLAB Function  TreatAsAtomicUnit=on
  wires:
  deBiaser1/1(y) -> To Workspace3/1, Scope5/4  "simTime"
  deBiaser3/1(y) -> To Workspace1/1, Scope5/2  "time_diff"
  flightTime/1 -> Sum2/2, Sum1/2, deBiaser2/1(u)
  MATLAB Function1/1(WINDOWStimeSec) -> Sum1/1, deBiaser/1(u)  "windowsTime"
  deBiaser2/1(y) -> To Workspace2/1, Scope5/3  "AeroflightTime"
  deBiaser/1(y) -> Scope5/1, To Workspace/1  "windowsTime"
  Sum1/1 -> deBiaser3/1(u)  "Tdiff"
  Clock/1 -> Sum2/1, deBiaser1/1(u)  "simtime"
  Sum2/1 -> deBiaser4/1(u)  "Tdiff"
  deBiaser4/1(y) -> To Workspace4/1, Scope5/5  "time_diff_sim"

== system model_16_09_22/ComputeError/ToWorkspace1 ==
  plane_coord_nwu : Inport
  MATLAB Function2 : MATLAB Function  TreatAsAtomicUnit=on
  To Workspace10 : ToWorkspace  VariableName=PosAircraftYnwu  SaveFormat=Structure  SampleTime=-1
  To Workspace8 : ToWorkspace  VariableName=PosAircraftXnwu  SaveFormat=Structure  SampleTime=-1
  To Workspace9 : ToWorkspace  VariableName=PosAircraftZnwu  SaveFormat=Structure  SampleTime=-1
  wires:
  MATLAB Function2/2(posAircraftY) -> To Workspace10/1  "posAircraftYnwu"
  MATLAB Function2/3(posAircraftZ) -> To Workspace9/1  "posAircraftZnwu"
  MATLAB Function2/1(posAircraftX) -> To Workspace8/1  "posAircraftXnwu"
  plane_coord_nwu/1 -> MATLAB Function2/1(posAircraft)

== system model_16_09_22/ComputeError/ToWorkspace2 ==
  min_coord_path_clock : Inport
  MATLAB Function1 : MATLAB Function  TreatAsAtomicUnit=on
  To Workspace5 : ToWorkspace  VariableName=coordclockovertimeZ  SaveFormat=Structure With Time  SampleTime=-1
  To Workspace6 : ToWorkspace  VariableName=coordclockovertimeX  SaveFormat=Structure With Time  SampleTime=-1
  To Workspace7 : ToWorkspace  VariableName=coordclockovertimeY  SaveFormat=Structure With Time  SampleTime=-1
  wires:
  MATLAB Function1/2(coordclockY) -> To Workspace7/1  "coordclockY"
  MATLAB Function1/3(coordclockZ) -> To Workspace5/1  "coordclockZ"
  MATLAB Function1/1(coordclockX) -> To Workspace6/1  "coordclockX"
  min_coord_path_clock/1 -> MATLAB Function1/1(coordclock)

== system model_16_09_22/ComputeError/ToWorkspace3 ==
  intersection_point : Inport
  MATLAB Function : MATLAB Function  TreatAsAtomicUnit=on
  To Workspace2 : ToWorkspace  VariableName=intersectionPointX  SaveFormat=Structure  SampleTime=-1
  To Workspace3 : ToWorkspace  VariableName=intersectionPointZ  SaveFormat=Structure  SampleTime=-1
  To Workspace4 : ToWorkspace  VariableName=intersectionPointY  SaveFormat=Structure  SampleTime=-1
  wires:
  MATLAB Function/3(intersectionPointhZ) -> To Workspace3/1  "intersectionPointz"
  MATLAB Function/2(intersectionPointY) -> To Workspace4/1  "intersectionPointY"
  MATLAB Function/1(intersectionPointX) -> To Workspace2/1  "intersectionPointX"
  intersection_point/1 -> MATLAB Function/1(intersectionPoint)

== system model_16_09_22/ComputeError/ToWorkspace4 ==
  aircraft2path : Inport
  MATLAB Function1 : MATLAB Function  TreatAsAtomicUnit=on
  To Workspace5 : ToWorkspace  VariableName=aircraft2pathZ  SaveFormat=Structure With Time  SampleTime=-1
  To Workspace6 : ToWorkspace  VariableName=aircraft2pathX  SaveFormat=Structure With Time  SampleTime=-1
  To Workspace7 : ToWorkspace  VariableName=aircraft2pathY  SaveFormat=Structure With Time  SampleTime=-1
  wires:
  MATLAB Function1/2(aircraft2pathY) -> To Workspace7/1  "aircraft2pathY"
  MATLAB Function1/3(aircraft2pathZ) -> To Workspace5/1  "aircraft2pathZ"
  MATLAB Function1/1(aircraft2pathX) -> To Workspace6/1  "aircraft2pathX"
  aircraft2path/1 -> MATLAB Function1/1(aircraft2path)

== system model_16_09_22/Controllers/IHA ==
  torqueRollXtrim : Inport
  torquePitchXtrim : Inport  Port=2
  LTI System2 : cstblocks/LTI System  sys=TDpitch  IC=[]
  LTI System3 : cstblocks/LTI System  sys=TDroll  IC=[]
  Out1 : Outport
  Out2 : Outport  Port=2
  wires:
  torquePitchXtrim/1 -> LTI System2/1
  torqueRollXtrim/1 -> LTI System3/1
  LTI System3/1 -> Out1/1
  LTI System2/1 -> Out2/1

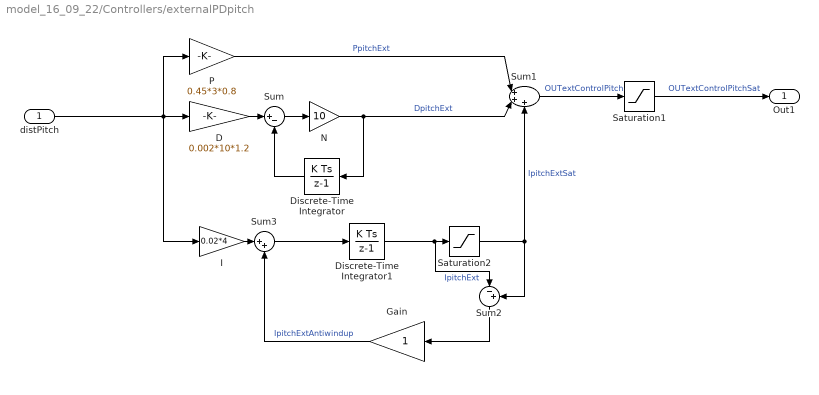
== system model_16_09_22/Controllers/externalPDpitch ==
  distPitch : Inport
  D : Gain  Gain=0.002*10*1.2
  Discrete-Time Integrator : DiscreteIntegrator  SampleTime=-1  ICPrevOutput=DiscIntNeverNeededParam  ICPrevScaledInput=DiscIntNeverNeededParam
  Discrete-Time Integrator1 : DiscreteIntegrator  SampleTime=-1  ICPrevOutput=DiscIntNeverNeededParam  ICPrevScaledInput=DiscIntNeverNeededParam
  Gain : Gain
  I : Gain  Gain=0.02*4
  N : Gain  Gain=10
  P : Gain  Gain=0.45*3*0.8
  Saturation1 : Saturate  UpperLimit=40  LowerLimit=-40
  Saturation2 : Saturate  UpperLimit=3  LowerLimit=-3
  Sum : Sum  Inputs=|+-
  Sum1 : Sum  Inputs=|+++
  Sum2 : Sum  Inputs=|-+
  Sum3 : Sum  Inputs=|++
  Out1 : Outport
  wires:
  D/1 -> Sum/1
  Sum/1 -> N/1
  Discrete-Time Integrator/1 -> Sum/2
  N/1 -> Sum1/2, Discrete-Time Integrator/1  "DpitchExt"
  P/1 -> Sum1/1  "PpitchExt"
  distPitch/1 -> D/1, I/1, P/1
  Discrete-Time Integrator1/1 -> Sum2/1, Saturation2/1  "IpitchExt"
  I/1 -> Sum3/1
  Sum2/1 -> Gain/1
  Sum3/1 -> Discrete-Time Integrator1/1
  Sum1/1 -> Saturation1/1  "OUTextControlPitch"
  Saturation1/1 -> Out1/1  "OUTextControlPitchSat"
  Saturation2/1 -> Sum1/3, Sum2/2  "IpitchExtSat"
  Gain/1 -> Sum3/2  "IpitchExtAntiwindup"

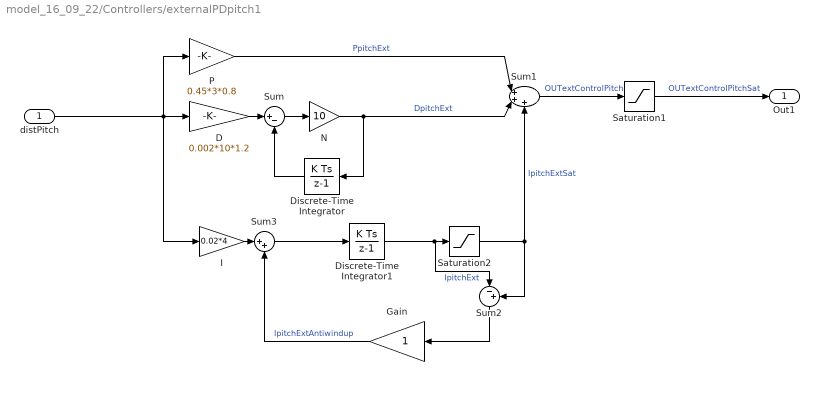
== system model_16_09_22/Controllers/externalPDpitch1 ==
  distPitch : Inport
  D : Gain  Gain=0.002*10*1.2
  Discrete-Time Integrator : DiscreteIntegrator  SampleTime=-1  ICPrevOutput=DiscIntNeverNeededParam  ICPrevScaledInput=DiscIntNeverNeededParam
  Discrete-Time Integrator1 : DiscreteIntegrator  SampleTime=-1  ICPrevOutput=DiscIntNeverNeededParam  ICPrevScaledInput=DiscIntNeverNeededParam
  Gain : Gain
  I : Gain  Gain=0.02*4
  N : Gain  Gain=10
  P : Gain  Gain=0.45*3*0.8
  Saturation1 : Saturate  UpperLimit=40  LowerLimit=-40
  Saturation2 : Saturate  UpperLimit=3  LowerLimit=-3
  Sum : Sum  Inputs=|+-
  Sum1 : Sum  Inputs=|+++
  Sum2 : Sum  Inputs=|-+
  Sum3 : Sum  Inputs=|++
  Out1 : Outport
  wires:
  D/1 -> Sum/1
  Sum/1 -> N/1
  Discrete-Time Integrator/1 -> Sum/2
  N/1 -> Sum1/2, Discrete-Time Integrator/1  "DpitchExt"
  P/1 -> Sum1/1  "PpitchExt"
  distPitch/1 -> D/1, I/1, P/1
  Discrete-Time Integrator1/1 -> Sum2/1, Saturation2/1  "IpitchExt"
  I/1 -> Sum3/1
  Sum2/1 -> Gain/1
  Sum3/1 -> Discrete-Time Integrator1/1
  Sum1/1 -> Saturation1/1  "OUTextControlPitch"
  Saturation1/1 -> Out1/1  "OUTextControlPitchSat"
  Saturation2/1 -> Sum1/3, Sum2/2  "IpitchExtSat"
  Gain/1 -> Sum3/2  "IpitchExtAntiwindup"

== system model_16_09_22/Controllers/externalPDroll ==
  distRollFilteredOld : Inport
  D : Gain  Gain=0.6*2
  Discrete-Time Integrator : DiscreteIntegrator  SampleTime=-1  ICPrevOutput=DiscIntNeverNeededParam  ICPrevScaledInput=DiscIntNeverNeededParam
  N : Gain
  P : Gain  Gain=0.2*1.5
  Saturation1 : Saturate  UpperLimit=40  LowerLimit=-40
  Sum : Sum  Inputs=|+-
  Sum1 : Sum  Inputs=|++
  Out1 : Outport
  wires:
  Sum/1 -> N/1
  N/1 -> Sum1/2, Discrete-Time Integrator/1  "DextRollOld"
  D/1 -> Sum/1
  distRollFilteredOld/1 -> P/1, D/1
  Saturation1/1 -> Out1/1  "OUTextControlRollSatOld"
  Sum1/1 -> Saturation1/1  "OUTextControlRollOld"
  Discrete-Time Integrator/1 -> Sum/2
  P/1 -> Sum1/1  "PextRollOld"

== system model_16_09_22/Controllers/externalPDroll1 ==
  distRollFiltered : Inport
  D : Gain  Gain=0.6*2
  Discrete-Time Integrator : DiscreteIntegrator  SampleTime=-1  ICPrevOutput=DiscIntNeverNeededParam  ICPrevScaledInput=DiscIntNeverNeededParam
  N : Gain
  P : Gain  Gain=0.2*1.5
  Saturation1 : Saturate  UpperLimit=40  LowerLimit=-40
  Sum : Sum  Inputs=|+-
  Sum1 : Sum  Inputs=|++
  Out1 : Outport
  wires:
  P/1 -> Sum1/1  "PextRoll"
  Discrete-Time Integrator/1 -> Sum/2
  Sum1/1 -> Saturation1/1  "OUTextControlRoll"
  Saturation1/1 -> Out1/1  "OUTextControlRollSat"
  distRollFiltered/1 -> D/1, P/1
  D/1 -> Sum/1
  N/1 -> Discrete-Time Integrator/1, Sum1/2  "DextRoll"
  Sum/1 -> N/1

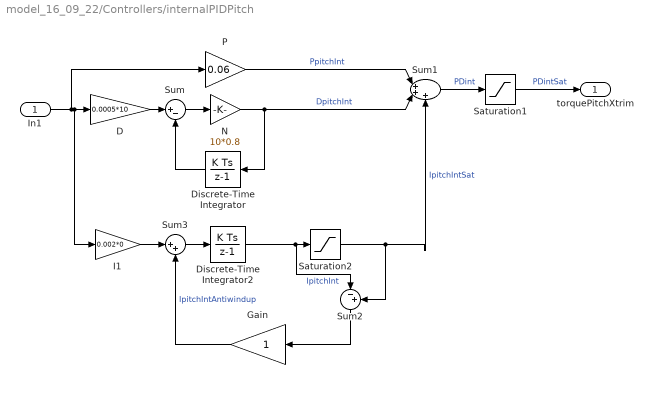
== system model_16_09_22/Controllers/internalPIDPitch ==
  In1 : Inport
  D : Gain  Gain=0.0005*10
  Discrete-Time Integrator : DiscreteIntegrator  SampleTime=-1  ICPrevOutput=DiscIntNeverNeededParam  ICPrevScaledInput=DiscIntNeverNeededParam
  Discrete-Time Integrator2 : DiscreteIntegrator  SampleTime=-1  ICPrevOutput=DiscIntNeverNeededParam  ICPrevScaledInput=DiscIntNeverNeededParam
  Gain : Gain
  I1 : Gain  Gain=0.002*0
  N : Gain  Gain=10*0.8
  P : Gain  Gain=0.06
  Saturation1 : Saturate  UpperLimit=1  LowerLimit=-1
  Saturation2 : Saturate  UpperLimit=1  LowerLimit=-1
  Sum : Sum  Inputs=|+-
  Sum1 : Sum  Inputs=|+++
  Sum2 : Sum  Inputs=|-+
  Sum3 : Sum  Inputs=|++
  torquePitchXtrim : Outport
  wires:
  D/1 -> Sum/1
  Sum/1 -> N/1
  Discrete-Time Integrator/1 -> Sum/2
  N/1 -> Sum1/2, Discrete-Time Integrator/1  "DpitchInt"
  P/1 -> Sum1/1  "PpitchInt"
  Saturation1/1 -> torquePitchXtrim/1  "PDintSat"
  Sum1/1 -> Saturation1/1  "PDint"
  In1/1 -> P/1, I1/1, D/1
  I1/1 -> Sum3/1
  Discrete-Time Integrator2/1 -> Sum2/1, Saturation2/1  "IpitchInt"
  Sum2/1 -> Gain/1
  Gain/1 -> Sum3/2  "IpitchIntAntiwindup"
  Sum3/1 -> Discrete-Time Integrator2/1
  Saturation2/1 -> Sum1/3, Sum2/2  "IpitchIntSat"

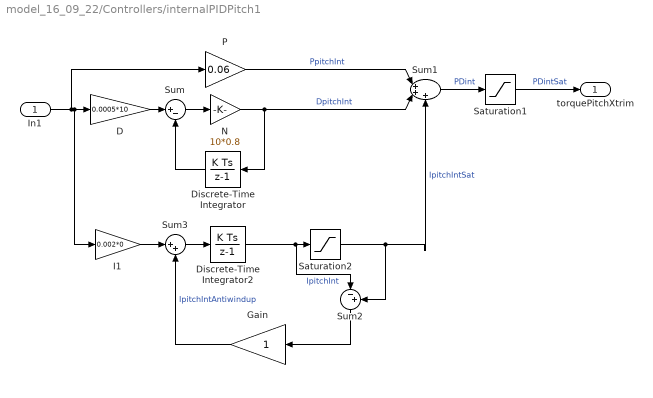
== system model_16_09_22/Controllers/internalPIDPitch1 ==
  In1 : Inport
  D : Gain  Gain=0.0005*10
  Discrete-Time Integrator : DiscreteIntegrator  SampleTime=-1  ICPrevOutput=DiscIntNeverNeededParam  ICPrevScaledInput=DiscIntNeverNeededParam
  Discrete-Time Integrator2 : DiscreteIntegrator  SampleTime=-1  ICPrevOutput=DiscIntNeverNeededParam  ICPrevScaledInput=DiscIntNeverNeededParam
  Gain : Gain
  I1 : Gain  Gain=0.002*0
  N : Gain  Gain=10*0.8
  P : Gain  Gain=0.06
  Saturation1 : Saturate  UpperLimit=1  LowerLimit=-1
  Saturation2 : Saturate  UpperLimit=1  LowerLimit=-1
  Sum : Sum  Inputs=|+-
  Sum1 : Sum  Inputs=|+++
  Sum2 : Sum  Inputs=|-+
  Sum3 : Sum  Inputs=|++
  torquePitchXtrim : Outport
  wires:
  D/1 -> Sum/1
  Sum/1 -> N/1
  Discrete-Time Integrator/1 -> Sum/2
  N/1 -> Sum1/2, Discrete-Time Integrator/1  "DpitchInt"
  P/1 -> Sum1/1  "PpitchInt"
  Saturation1/1 -> torquePitchXtrim/1  "PDintSat"
  Sum1/1 -> Saturation1/1  "PDint"
  In1/1 -> P/1, I1/1, D/1
  I1/1 -> Sum3/1
  Discrete-Time Integrator2/1 -> Sum2/1, Saturation2/1  "IpitchInt"
  Sum2/1 -> Gain/1
  Gain/1 -> Sum3/2  "IpitchIntAntiwindup"
  Sum3/1 -> Discrete-Time Integrator2/1
  Saturation2/1 -> Sum1/3, Sum2/2  "IpitchIntSat"

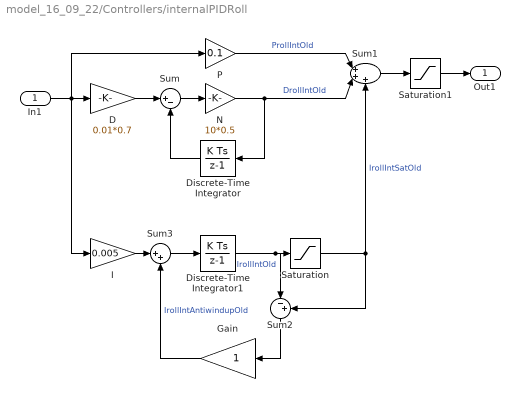
== system model_16_09_22/Controllers/internalPIDRoll ==
  In1 : Inport
  D : Gain  Gain=0.01*0.7
  Discrete-Time Integrator : DiscreteIntegrator  SampleTime=-1  ICPrevOutput=DiscIntNeverNeededParam  ICPrevScaledInput=DiscIntNeverNeededParam
  Discrete-Time Integrator1 : DiscreteIntegrator  SampleTime=-1  ICPrevOutput=DiscIntNeverNeededParam  ICPrevScaledInput=DiscIntNeverNeededParam
  Gain : Gain
  I : Gain  Gain=0.005
  N : Gain  Gain=10*0.5
  P : Gain  Gain=0.1
  Saturation : Saturate
  Saturation1 : Saturate  UpperLimit=1  LowerLimit=-1
  Sum : Sum  Inputs=|+-
  Sum1 : Sum  Inputs=|+++
  Sum2 : Sum  Inputs=|-+
  Sum3 : Sum  Inputs=|++
  Out1 : Outport
  wires:
  P/1 -> Sum1/1  "ProllIntOld"
  In1/1 -> P/1, I/1, D/1
  Sum/1 -> N/1
  D/1 -> Sum/1
  N/1 -> Sum1/2, Discrete-Time Integrator/1  "DrollIntOld"
  I/1 -> Sum3/1
  Saturation1/1 -> Out1/1
  Discrete-Time Integrator/1 -> Sum/2
  Sum1/1 -> Saturation1/1
  Sum2/1 -> Gain/1
  Gain/1 -> Sum3/2  "IrollIntAntiwindupOld"
  Saturation/1 -> Sum2/2, Sum1/3  "IrollIntSatOld"
  Discrete-Time Integrator1/1 -> Sum2/1, Saturation/1  "IrollIntOld"
  Sum3/1 -> Discrete-Time Integrator1/1

== system model_16_09_22/Controllers/internalPIDRoll1 ==
  In1 : Inport
  D : Gain  Gain=0.01*0.7
  Discrete-Time Integrator : DiscreteIntegrator  SampleTime=-1  ICPrevOutput=DiscIntNeverNeededParam  ICPrevScaledInput=DiscIntNeverNeededParam
  Discrete-Time Integrator1 : DiscreteIntegrator  SampleTime=-1  ICPrevOutput=DiscIntNeverNeededParam  ICPrevScaledInput=DiscIntNeverNeededParam
  Gain : Gain
  I : Gain  Gain=0.005
  N : Gain  Gain=10*0.5
  P : Gain  Gain=0.1
  Saturation : Saturate
  Saturation1 : Saturate  UpperLimit=1  LowerLimit=-1
  Sum : Sum  Inputs=|+-
  Sum1 : Sum  Inputs=|+++
  Sum2 : Sum  Inputs=|-+
  Sum3 : Sum  Inputs=|++
  Out1 : Outport
  wires:
  Sum3/1 -> Discrete-Time Integrator1/1
  Discrete-Time Integrator1/1 -> Saturation/1, Sum2/1  "IrollInt"
  Saturation/1 -> Sum1/3, Sum2/2  "IrollIntSat"
  Gain/1 -> Sum3/2  "IrollIntAntiwindup"
  Sum2/1 -> Gain/1
  Sum1/1 -> Saturation1/1
  Discrete-Time Integrator/1 -> Sum/2
  Saturation1/1 -> Out1/1
  I/1 -> Sum3/1
  N/1 -> Discrete-Time Integrator/1, Sum1/2  "DrollInt"
  D/1 -> Sum/1
  Sum/1 -> N/1
  In1/1 -> D/1, I/1, P/1
  P/1 -> Sum1/1  "ProllInt"

== system model_16_09_22/MagnitudeReceive/axis 1 ==
  In1 : Inport
  In2 : Inport  Port=2
  Enable : EnablePort
  slider scaling constant : Gain  Gain=1690
  Out1 : Outport
  Out2 : Outport  Port=2
  wires:
  slider scaling constant/1 -> Out1/1
  In1/1 -> slider scaling constant/1
  In2/1 -> Out2/1

== system model_16_09_22/MagnitudeReceive/axis 2 ==
  In1 : Inport
  In2 : Inport  Port=2
  Enable : EnablePort
  slider scaling constant : Gain  Gain=1680
  Out1 : Outport
  Out2 : Outport  Port=2
  wires:
  In1/1 -> slider scaling constant/1
  slider scaling constant/1 -> Out1/1
  In2/1 -> Out2/1

== system model_16_09_22/MagnitudeReceive/axis 3 ==
  In1 : Inport
  Enable : EnablePort
  dial  scaling constant : Gain  Gain=1995
  Out1 : Outport
  wires:
  dial  scaling constant/1 -> Out1/1
  In1/1 -> dial  scaling constant/1

== system model_16_09_22/MagnitudeReceive/logMotorTorque ==
  motorTorqueVector : Inport
  MATLAB Function1 : MATLAB Function  TreatAsAtomicUnit=on
  To Workspace1 : ToWorkspace  VariableName=motorTorqueY  SaveFormat=Structure With Time  SampleTime=-1
  To Workspace2 : ToWorkspace  VariableName=motorTorqueX  SaveFormat=Structure With Time  SampleTime=-1
  wires:
  MATLAB Function1/2(motorTorqueY) -> To Workspace1/1  "stickDeflectionYScaled"
  MATLAB Function1/1(motorTorqueX) -> To Workspace2/1  "stickDeflectionXScaled"
  motorTorqueVector/1 -> MATLAB Function1/1(motorTorqueVector)

== system model_16_09_22/MagnitudeReceive/logStickDeflection ==
  stickDeflectionScaled : Inport
  MATLAB Function1 : MATLAB Function  TreatAsAtomicUnit=on
  To Workspace6 : ToWorkspace  VariableName=stickDeflectionZ  SaveFormat=Structure With Time  SampleTime=-1
  To Workspace7 : ToWorkspace  VariableName=stickDeflectionX  SaveFormat=Structure With Time  SampleTime=-1
  To Workspace8 : ToWorkspace  VariableName=stickDeflectionY  SaveFormat=Structure With Time  SampleTime=-1
  wires:
  stickDeflectionScaled/1 -> MATLAB Function1/1(stickDeflection)
  MATLAB Function1/2(stickDeflectionY) -> To Workspace8/1  "stistickDeflectionYScaled"
  MATLAB Function1/3(stickDeflectionZ) -> To Workspace6/1  "stickDeflectionZScaled"
  MATLAB Function1/1(stickDeflectionX) -> To Workspace7/1  "stickDeflectionXScaled"

== matlab function model_16_09_22/Controllers/roll ==
  data: intersection2path input; s input; dist output
function dist = fcn(intersection2path, s) 
    %BUILDING ROLL COMMAND
    %rollio a posizione laterale
    %distXY = sqrt((min_valid_aircraft2path(1)^2) + (min_valid_aircraft2path(2)^2)); 

    x = norm(intersection2path);
      
    %i want set a sign for this lenght   
    if ((norm(intersection2path)> 0) && (s > 0))
        dist = - x ;
    elseif ((norm(intersection2path)> 0) && (s < 0))
        dist = x ;
    else
        dist = 0;
    end

== matlab function model_16_09_22/CoordinatesConversions/MATLAB Function3 ==
  data: lon input; lonDeg output; lat input; latDeg output
function [lonDeg, latDeg] = fcn(lon, lat)
        lonDeg = rad2deg(lon);
        latDeg = rad2deg(lat);
end

== matlab function model_16_09_22/CoordinatesConversions/MATLAB Function2 ==
  data: coord_0_ecef parameter; coord_ecef input; plane_coord_nwu output; coord_ecef_aerofly input; plane_coord_nwu_aerofly output; RotationMatrix_NWU2ECEF parameter; alt input
% --------------------------------------------------------------------------------#
%    ecef2nWU(): coordinate transformation from ECEF system to NWU system         #
% --------------------------------------------------------------------------------#

function [plane_coord_nwu, plane_coord_nwu_aerofly]  = ecef2nwu(coord_0_ecef, coord_ecef, coord_ecef_aerofly, RotationMatrix_NWU2ECEF, alt)

     %---Rotatiting the distance vector-----------------------------------% 
     %transpose vector to compute product with matrix
     vector_ref1 = (coord_ecef - coord_0_ecef).'; 
     %transpose final vector again to have an orizontal vector
     plane_coord_nwu = ((RotationMatrix_NWU2ECEF)\(vector_ref1)).';
     %FORZA BRUTA
     %plane_coord_nwu(3) = data;
     %plane_coord_nwu =  (RotationMatrix_ECEF2NWU * (vector_ref1)).';
     %---Rotatiting the distance vector-----------------------------------% 
     %---between the center of the earth and the local frame--------------%
     %---USING AEROFLY ECEF COORDINATES-----------------------------------%
     vector_ref1 = (coord_ecef_aerofly - coord_0_ecef).';
     plane_coord_nwu_aerofly = ((RotationMatrix_NWU2ECEF)\(vector_ref1)).';
     %FORZA BRUTA
     plane_coord_nwu_aerofly(3) = alt;
end

== matlab function model_16_09_22/Controllers/Pitch ==
  data: h input; distPitch output
function distPitch = fcn(h)
    %PITCH   
    %distZ = abs(min_valid_aircraft2path(3));
    deadZoneZ = 0;  %[m]
    
    y = h ;
    
    if ((abs(h) > deadZoneZ) && (h > 0))
        errorheight = abs(abs(y) - deadZoneZ);
    elseif ((abs(h) > deadZoneZ) && (h < 0))
        errorheight = - abs(abs(y) - deadZoneZ); %y<0
    else
        errorheight = 0;
    end
    
    distPitch = errorheight;

== matlab function model_16_09_22/ComputeError/computeError ==
  data: plane_coord_nwu input; intersection2path output; intersection_point output; min_valid_tangent input; h output; norm_min_valid_aircraft2path input; min_valid_coord_clock input; s output; t output; first_vector output; second_vector output; third_vector output

function [intersection2path, intersection_point, h, s, t,...
          first_vector, second_vector, third_vector] = compute_feedback(plane_coord_nwu, min_valid_tangent, ...
          norm_min_valid_aircraft2path, min_valid_coord_clock)
    
   %taking tangent and coordinates of the pathClock
   %corresponding to the min valid index found
    pos_airplane = plane_coord_nwu;
    min_valid_tangent = min_valid_tangent/norm(min_valid_tangent);
    
    % rotation to get the orto vector
    rotmat = [0,1 ; -1,0];

    ot_xy = rotmat * [min_valid_tangent(1); min_valid_tangent(2)] ;
    ot_xyz = [ot_xy(1), ot_xy(2), 0]; % set z component to 0
    orthotangent = ot_xyz / norm(ot_xyz);
    cross_vector = cross(orthotangent, min_valid_tangent);
    
       
    %building our plane with the three vectors found  
    %all vectors are normalized
    first_vector = orthotangent; %/norm(orthotangent);
    second_vector = min_valid_tangent; %/norm(tangent);
    third_vector = cross_vector; %/norm(cross_vector)
    
    
    %aircraft2path = - (pos_airplane - coord_clock_on_path)
    %known_value = (pos_airplane - coord_clock).'
    known_value = - norm_min_valid_aircraft2path.'; 
        
    A = [first_vector(1), second_vector(1), third_vector(1);
         first_vector(2), second_vector(2), third_vector(2);
         first_vector(3), second_vector(3), third_vector(3);];

    solutions_vector = A\known_value; %inv(A)*known_value; 
    s = solutions_vector(1);
    t = solutions_vector(2);
    h = solutions_vector(3);
    intersection_point = pos_airplane - h*third_vector;
    intersection2path = norm(intersection_point - min_valid_coord_clock); %ATTENZIONE A COORD CLOCK 

end
